simulink model "Commande_de_modele"  (R2023b)
settings: Solver=FixedStepAuto  StartTime=0.0  StopTime=1  FixedStep=1e-5  RelTol=1e-3
InitFcn:
  | C=4000e-6;
  | L=40e-3;
  | R=10;
  | E=12;
  | f=1e4;
settings Model: Creator=lenovo  LastModifiedBy=lenovo

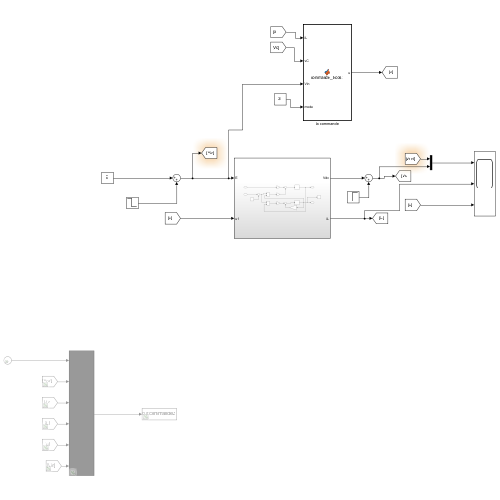
[thumbnail: Simulink's stored preview of the top-level diagram]
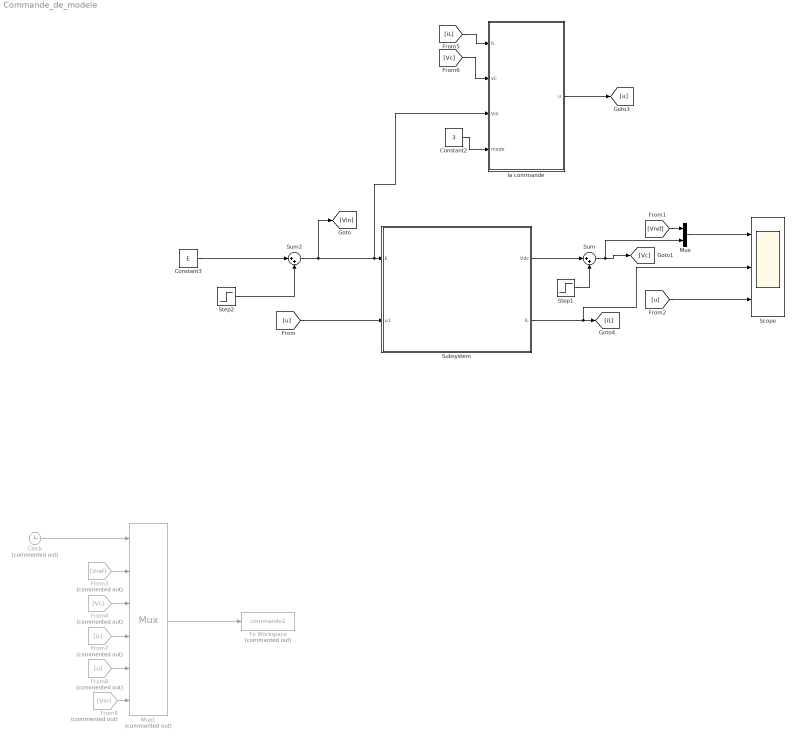
== system Commande_de_modele ==
  Clock : Clock  Commented=on
      settings: Decimation=1e5
  Constant2 : Constant  Value=3
  Constant3 : Constant  Value=E
  From3 : From  Commented=on  GotoTag=Vref
  From4 : From  Commented=on  GotoTag=Vc
  From7 : From  Commented=on  GotoTag=iL
  From8 : From  Commented=on  GotoTag=u
  From9 : From  Commented=on  GotoTag=Vin
  Mux : Mux  Inputs=2
  Mux1 : Mux  Commented=on  Inputs=6
  Scope : Scope  NumInputPorts=3
  Step1 : Step  Time=0.01  After=0  SampleTime=0
  Step2 : Step  Time=0.5  After=-3  SampleTime=0
  Subsystem : Subsystem
  Sum : Sum  Inputs=|++
  Sum2 : Sum  Inputs=|++
  To Workspace : ToWorkspace  Commented=on  VariableName=commande2  SampleTime=-1
      settings: Save2DSignal=2-D array (concatenate along first dimension)
  la commande : MATLAB Function  TreatAsAtomicUnit=on
  wires:
  la commande/1(u) -> [u]
  [iL] -> la commande/1(iL)
  [Vc] -> la commande/2(vC)
  Constant2/1 -> la commande/4(mode)
  [u] -> Subsystem/2(u1)
  Subsystem/2(iL) -> Scope/2, [iL]
  Mux/1 -> Scope/1
  [Vref] -> Mux/1
  [u] -> Scope/3
  Subsystem/1(Vdc) -> Sum/1
  Sum/1 -> Mux/2, [Vc]
  Step1/1 -> Sum/2
  Sum2/1 -> [Vin], la commande/3(Vin), Subsystem/1(E)
  Constant3/1 -> Sum2/1
  Step2/1 -> Sum2/2
  Mux1/1 -> To Workspace/1
  Clock/1 -> Mux1/1
  From3/1 -> Mux1/2
  From4/1 -> Mux1/3
  From7/1 -> Mux1/4
  From8/1 -> Mux1/5
  From9/1 -> Mux1/6

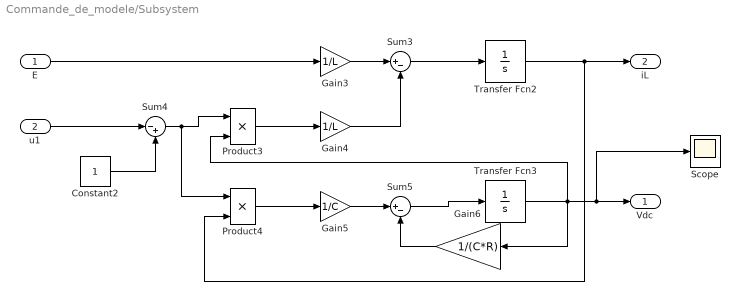
== system Commande_de_modele/Subsystem ==
  E : Inport
  u1 : Inport  Port=2
  Constant2 : Constant
  Gain3 : Gain  Gain=1/L
  Gain4 : Gain  Gain=1/L
  Gain5 : Gain  Gain=1/C
  Gain6 : Gain  Gain=1/(C*R)
  Product3 : Product
  Product4 : Product
  Scope : Scope
  Sum3 : Sum  Inputs=|+-
  Sum4 : Sum  Inputs=|-+
  Sum5 : Sum  Inputs=|+-
  Transfer Fcn2 : TransferFcn  Denominator=[1 0]
  Transfer Fcn3 : TransferFcn  Denominator=[1 0]
  Vdc : Outport
  iL : Outport  Port=2
  wires:
  E/1 -> Gain3/1
  Gain3/1 -> Sum3/1
  Gain4/1 -> Sum3/2
  u1/1 -> Sum4/1
  Constant2/1 -> Sum4/2
  Product3/1 -> Gain4/1
  Sum4/1 -> Product4/1, Product3/1
  Product4/1 -> Gain5/1
  Gain5/1 -> Sum5/1
  Gain6/1 -> Sum5/2
  Sum3/1 -> Transfer Fcn2/1
  Transfer Fcn2/1 -> Product4/2, iL/1
  Sum5/1 -> Transfer Fcn3/1
  Transfer Fcn3/1 -> Product3/2, Gain6/1, Scope/1, Vdc/1

== matlab function Commande_de_modele/la commande ==
  data: iL input; u output; vC input; Vin input; mode input
function u = commande_boost(iL, vC, Vin, mode)
% COMMANDE_BOOST
% Loi de commande non linéaire pour un convertisseur Boost.
%
% Entrées :
%   iL   : courant dans l'inductance (A)
%   vC   : tension de sortie (V)
%   Vin  : tension d'entrée instantanée (V)
%   mode : sélection de la loi de commande
%       1: commande à l'équilibre (u = u_eq)
%       2: Lyapunov : annulation complète de Vdot
%       3: Lyapunov : annulation des termes non stabilisants
%
% Sortie :
% u    : rapport cyclique


%% Paramètres de fonctionnement
R    = 10;    % résistance de charge (ohms)
Vref = 24;    % tension de sortie désirée (V)

%% 1) Point d'équilibre associé à Vref
u_eq  = 1 - Vin./Vref;      % duty à l'équilibre
iL_eq = Vref.^2./(R*Vin);   % courant inductif à l'équilibre
vC_eq = Vref;               % tension de sortie à l'équilibre

%% 2) Changement de Variables 
tilde_iL = iL - iL_eq;
tilde_vC = vC - vC_eq;

% Le terme non stable
w = vC_eq*tilde_iL - iL_eq*tilde_vC;

%% 3) Paramètres des lois de commande
alpha1 = 50;    % gain Lyapunov (commande 2) sur tilde_iL^2
alpha2 = 1.0;   % gain Lyapunov (commande 2) sur tilde_vC^2
k      = 0.5;   % gain Lyapunov (commande 3) sur w

%% 4) Sélection de la loi de commande
switch mode
    
    case 1
        % Mode 1 : duty simplement fixé à la valeur d'équilibre
        u = u_eq;
        
    case 2
        % Mode 2 : annulation complète de Vdot
        
        num = -alpha1*tilde_iL.^2 - (alpha2 - 1/R).*tilde_vC.^2;
        
        if abs(w) < 1e-6
            % si le dénominateur est trop petit, on évite la division
            u = u_eq;
        else
            u = u_eq + num./w;
        end
       
    case 3
        % Mode 3 : annulation des seuls termes non stabilisants
     
        u = u_eq - k*w;
        
    otherwise
        % mode non reconnu : on se rabat sur la commande à l'équilibre
        u = u_eq;
end

%% 5) Saturation du duty dans l'intervalle physique
u = max(min(u, 0.95), 0.05);

end
